simulink model "EV_model_TEMPLATE_2025a"  (R2025a)
settings: Solver=FixedStepAuto  StartTime=0.0  StopTime=1180  FixedStep=0.1  MaxStep=1e-3  RelTol=1e-3
values from neighbouring files (symbols this model uses):
  A = 2.3750    (= 2.375)    [EV_parameters.m]
  Cd = 0.24    [EV_parameters.m]
  Cr = 0.01    [EV_parameters.m]
  g = 9.81    [EV_parameters.m]
  gear_r = 9.6    [EV_parameters.m]
  grad = cos(theta)    [EV_parameters.m]
  m = 2000    [EV_parameters.m]    (also in brakes.m = 18000; powergraph.m = 18000)
  Np = 100    [EV_parameters.m]
  Ns = 100    [EV_parameters.m]
  P_max = 70    [EV_parameters.m]
  rho = 1.225    [EV_parameters.m]
  Ro = 0.07    [Battery_parameters.m]    (also in EV_parameters.m = 0.03)
  Rw = 0.35    [EV_parameters.m]
  T_max = 400    [EV_parameters.m]
  theta = 0.312    [Calculations.m]    (also in EV_parameters.m = 0)
  Voc = 3    [EV_parameters.m]
libraries: autolibshared x1, drivingcycle_lib x1, simulink x1
settings Model: Creator=Ashwil Augustin  LastModifiedBy=91944
settings SolverCC: AlgebraicLoopSolver=TrustRegion
settings DataIOCC: ReturnWorkspaceOutputs=off
settings DebuggingCC: UnconnectedInputMsg=warning  UnconnectedOutputMsg=warning  UnconnectedLineMsg=warning  PregeneratedLibrarySubsystemCodeDiagnostic=none  ArithmeticOperatorsInVariantConditions=warning
settings ModelReferenceCC: EnableRefExpFcnMdlSchedulingChecks=on
settings SFSimCC: SimUseLocalCustomCode=off  CustomCodeUndefinedFunction=UseInterfaceOnly
settings RTWCC: RTWUseLocalCustomCode=off  GPUComputeCapability=3.5  DLArmComputeVersion=19.05

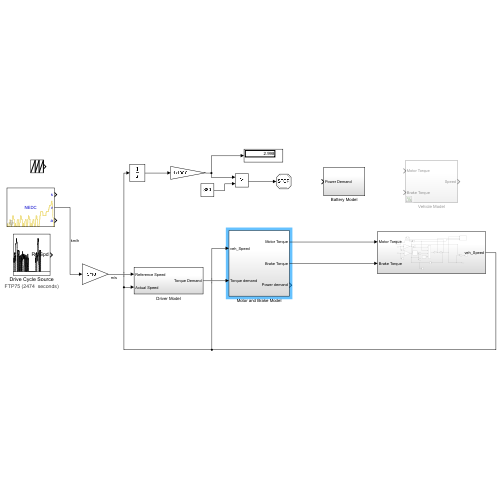
[thumbnail: Simulink's stored preview of the top-level diagram]
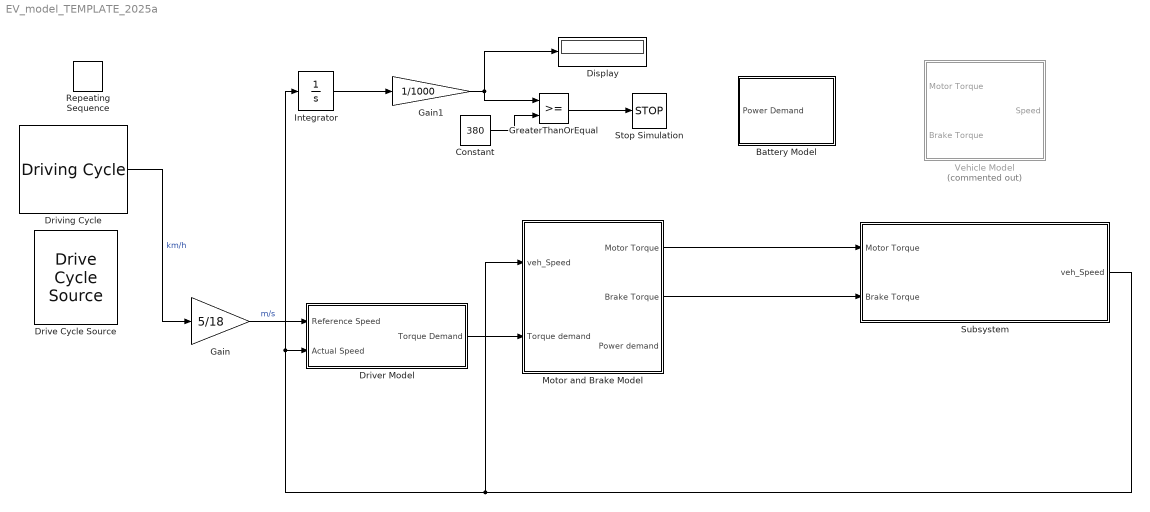
== system EV_model_TEMPLATE_2025a ==
  Battery Model : Subsystem
  Constant : Constant  Value=380
  Display : Display
  Drive Cycle Source : autolibshared/Drive Cycle Source  cycleVar=FTP75  fileVar=cycleFTP75.mat  tfinal="2474  seconds"  cycleRepeat=off  outAccPort=off  outGearPort=off  gearList=No gear data  t_wot1=5  xdot_woto=0  xdot_wot1=30  t_wot2=20  xdot_wot2=0  t_wotend=30  srcUnit=m/s  outUnit=m/s  srcAccUnit=m/s/s  outAccUnit=m/s^2  dt=0  aMode=2  faultOption=off  velBnd=2  velBndUnit=mph  inUnit=m/s  timeBnd=1  failOption=off  stopSim=off  maxFaultCnt=10  maxFaultTime=2  maxTotFaultTime=15  traceOption=off  dtTrace=1  traceWindow=10  lastDCname=FTP75  lastOutUnit=mph  lastDT=0  lastTB=1  lastSB=2  forceCalcBound=off
      settings: LibrarySourceBlock=vehdynlibscenario/Drive Cycle Source
  Driver Model : Subsystem
  Driving Cycle : drivingcycle_lib/Driving Cycle  CycleName=NEDC  CycleRepeatsForever=on
      settings: SourceProductName=Driving Cycle Blockset
  Gain : Gain  Gain=5/18
  Gain1 : Gain  Gain=1/1000
  GreaterThanOrEqual : RelationalOperator  OutDataTypeStr=boolean  RndMeth=Simplest  InputSameDT=off
  Integrator : Integrator
  Motor and Brake Model : Subsystem
  Repeating Sequence : simulink/Sources/Repeating Sequence  rep_seq_t=[0 2]  rep_seq_y=[0 2]
  Stop Simulation : Stop
  Subsystem : Subsystem
  Vehicle Model : Subsystem  Commented=on
  wires:
  Motor and Brake Model/1(Motor Torque) -> Subsystem/1("Motor Torque ")
  Driver Model/1(Torque Demand) -> Motor and Brake Model/2(Torque demand)
  Subsystem/1(veh_Speed) -> Motor and Brake Model/1(veh_Speed), Integrator/1, Driver Model/2(Actual Speed)
  Motor and Brake Model/2(Brake Torque) -> Subsystem/2(Brake Torque)
  Driving Cycle/2 -> Gain/1  "km/h"
  Gain/1 -> Driver Model/1(Reference Speed)  "m/s"
  Integrator/1 -> Gain1/1
  Constant/1 -> GreaterThanOrEqual/2
  GreaterThanOrEqual/1 -> Stop Simulation/1
  Gain1/1 -> GreaterThanOrEqual/1, Display/1

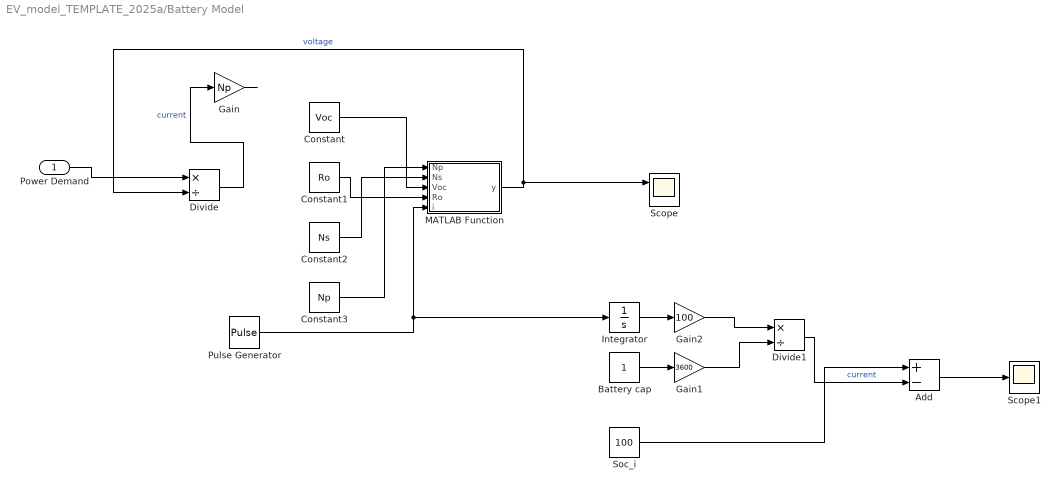
== system EV_model_TEMPLATE_2025a/Battery Model ==
  Power Demand : Inport
  Add : Sum  Inputs=+-
  Battery cap : Constant
  Constant : Constant  Value=Voc
  Constant1 : Constant  Value=Ro
  Constant2 : Constant  Value=Ns
  Constant3 : Constant  Value=Np
  Divide : Product  Inputs=*/
  Divide1 : Product  Inputs=*/
  Gain : Gain  Gain=Np
  Gain1 : Gain  Gain=3600
  Gain2 : Gain  Gain=100
  Integrator : Integrator
  MATLAB Function : MATLAB Function  TreatAsAtomicUnit=on
  Pulse Generator : DiscretePulseGenerator  PulseType=Time based  Period=10  PulseWidth=5
  Scope : Scope  NumInputPorts=2
      settings: ActiveDisplayYMinimum=2.96625  ActiveDisplayYMaximum=3.00375  DataLoggingVariableName=ScopeData2
  Scope1 : Scope
      settings: ActiveDisplayYMinimum=99.900032517604046  ActiveDisplayYMaximum=100.11119248089466  DataLoggingVariableName=ScopeData5
  Soc_i : Constant  Value=100
  wires:
  Constant3/1 -> MATLAB Function/1(Np)
  Constant2/1 -> MATLAB Function/2(Ns)
  Constant1/1 -> MATLAB Function/4(Ro)
  Constant/1 -> MATLAB Function/3(Voc)
  MATLAB Function/1(y) -> Divide/2, Scope/1  "voltage"
  Power Demand/1 -> Divide/1
  Divide/1 -> Gain/1  "current"
  Gain/1 -> ?
  Integrator/1 -> Gain2/1
  Battery cap/1 -> Gain1/1
  Gain2/1 -> Divide1/1
  Gain1/1 -> Divide1/2
  Soc_i/1 -> Add/1
  Divide1/1 -> Add/2  "current"
  Add/1 -> Scope1/1
  Pulse Generator/1 -> Integrator/1, MATLAB Function/5(i)

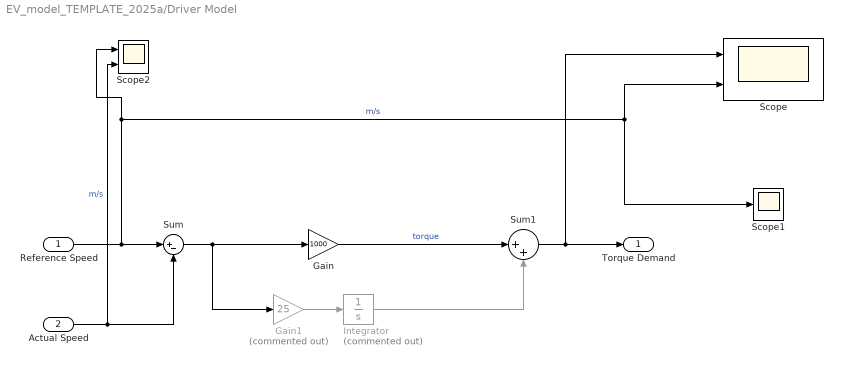
== system EV_model_TEMPLATE_2025a/Driver Model ==
  Reference Speed : Inport
  Actual Speed : Inport  Port=2
  Gain : Gain  Gain=1000
  Gain1 : Gain  Commented=on  Gain=25
  Integrator : Integrator  Commented=on
  Scope : Scope  NumInputPorts=2
      settings: ActiveDisplayYMinimum=-9.488488226261536  ActiveDisplayYMaximum=85.39639403635384  DataLoggingVariableName=ScopeData7
  Scope1 : Scope
      settings: ActiveDisplayYMinimum=-1  ActiveDisplayYMaximum=1  DataLoggingVariableName=ScopeData14
  Scope2 : Scope  NumInputPorts=2
      settings: ActiveDisplayYMinimum=3.7832627004980979  ActiveDisplayYMaximum=3.895862810225073  DataLoggingVariableName=ScopeData15
  Sum : Sum  Inputs=|+-
  Sum1 : Sum  Inputs=|++
  Torque Demand : Outport  VectorParamsAs1DForOutWhenUnconnected=off
  wires:
  Reference Speed/1 -> Scope2/1, Scope1/1, Scope/2, Sum/1  "m/s"
  Actual Speed/1 -> Scope2/2, Sum/2  "m/s"
  Sum/1 -> Gain1/1, Gain/1
  Gain/1 -> Sum1/1  "torque"
  Sum1/1 -> Scope/1, Torque Demand/1
  Integrator/1 -> Sum1/2
  Gain1/1 -> Integrator/1

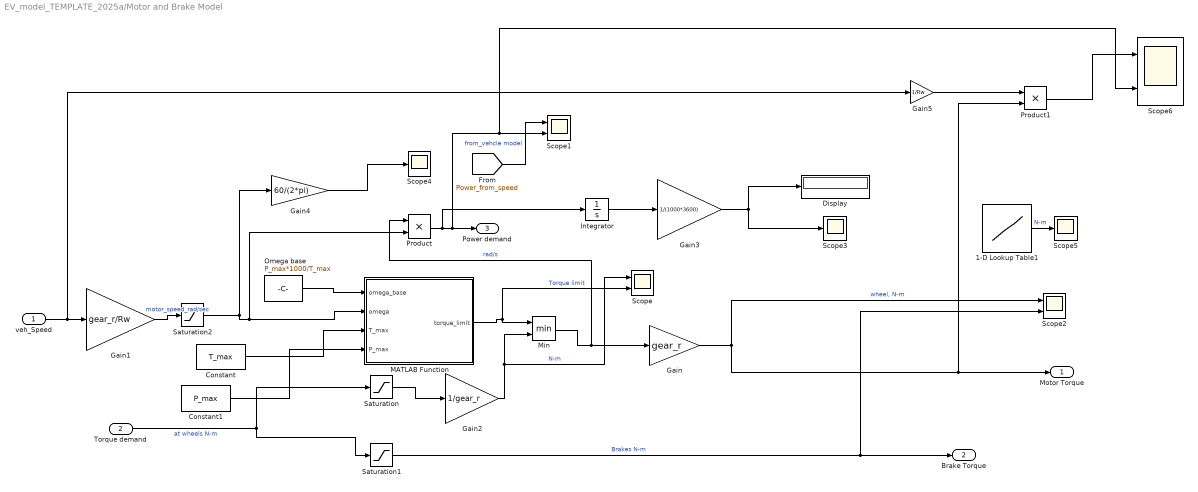
== system EV_model_TEMPLATE_2025a/Motor and Brake Model ==
  veh_Speed : Inport
  Torque demand : Inport  Port=2
  1-D Lookup Table1 : Lookup_n-D  NumberOfTableDimensions=1  BreakpointsForDimension1=[0,0.5*(70000/400), (70000/400), 2*(70000/400), 3*70000/400, 4*70000/400 ]  Table=[400,400, 400, 400/2, 400/3, 400/4]  InternalRulePriority=Speed  RndMeth=Simplest
  Constant : Constant  Value=T_max
  Constant1 : Constant  Value=P_max
  Display : Display
  Gain : Gain  Gain=gear_r
  Gain1 : Gain  Gain=gear_r/Rw
  Gain2 : Gain  Gain=1/gear_r
  Gain3 : Gain  Gain=1/(1000*3600)
  Gain4 : Gain  Gain=60/(2*pi)
  Gain5 : Gain  Gain=1/Rw
  Integrator : Integrator
  MATLAB Function : MATLAB Function  TreatAsAtomicUnit=on
  Min : MinMax  Inputs=2
  Omega base : Constant  Value=P_max*1000/T_max
  Product : Product
  Product1 : Product
  Saturation : Saturate  UpperLimit=inf  LowerLimit=0
  Saturation1 : Saturate  UpperLimit=0  LowerLimit=-inf
  Saturation2 : Saturate  UpperLimit=16000*(2*pi/60)  LowerLimit=0
  Scope{,1..2,6} (4 alike) : Scope  NumInputPorts=2
      Scope settings: ActiveDisplayYMinimum=-5.4943840804841173  ActiveDisplayYMaximum=30.78226270566185  DataLoggingVariableName=ScopeData3
      Scope1 settings: ActiveDisplayYMinimum=-7885.4073770511395  ActiveDisplayYMaximum=37796.877105105457  DataLoggingVariableName=ScopeData12
      Scope2 settings: ActiveDisplayYMinimum=-34.343817209843884  ActiveDisplayYMaximum=309.09435488859503  DataLoggingVariableName=ScopeData8
      Scope6 settings: ActiveDisplayYMinimum=-1  ActiveDisplayYMaximum=1  DataLoggingVariableName=ScopeData18
  Scope3 : Scope
      settings: ActiveDisplayYMinimum=-12.059544490137064  ActiveDisplayYMaximum=30.683168127008138  DataLoggingVariableName=ScopeData13
  Scope4 : Scope
      settings: ActiveDisplayYMinimum=-1  ActiveDisplayYMaximum=1  DataLoggingVariableName=ScopeData17
  Scope5 : Scope
      settings: ActiveDisplayYMinimum=-1  ActiveDisplayYMaximum=1  DataLoggingVariableName=ScopeData6
  Motor Torque : Outport  VectorParamsAs1DForOutWhenUnconnected=off
  Brake Torque : Outport  Port=2  VectorParamsAs1DForOutWhenUnconnected=off
  Power demand : Outport  Port=3
  wires:
  Saturation1/1 -> Scope2/2, Brake Torque/1  "Brakes N-m"
  Torque demand/1 -> Saturation/1, Saturation1/1  "at wheels N-m"
  veh_Speed/1 -> Gain5/1, Gain1/1
  Gain1/1 -> Saturation2/1  "motor_speed_rad/sec"
  Gain2/1 -> Scope/1, Min/2  "N-m"
  Saturation/1 -> Gain2/1
  Gain/1 -> Product1/2, Motor Torque/1, Scope2/1  "wheel, N-m"
  Min/1 -> Product/1, Gain/1  "rad/s"
  Product/1 -> Integrator/1, Scope6/2, Scope1/2, Power demand/1
  Integrator/1 -> Gain3/1
  Gain3/1 -> Scope3/1, Display/1
  Gain4/1 -> Scope4/1
  Omega base/1 -> MATLAB Function/1(omega_base)
  Constant/1 -> MATLAB Function/3(T_max)
  Constant1/1 -> MATLAB Function/4(P_max)
  MATLAB Function/1(torque_limit) -> Scope/2, Min/1  "Torque limit"
  [Power_from_speed] -> Scope1/1  "from_vehcle model"
  Saturation2/1 -> Gain4/1, Product/2, MATLAB Function/2(omega)
  1-D Lookup Table1/1 -> Scope5/1  "N-m"
  Gain5/1 -> Product1/1
  Product1/1 -> Scope6/1

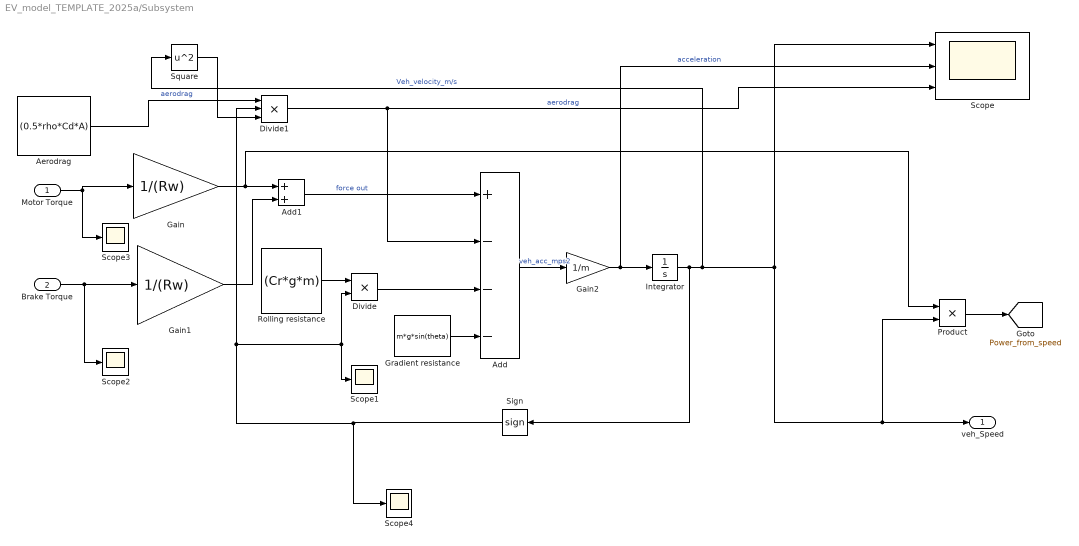
== system EV_model_TEMPLATE_2025a/Subsystem ==
  "Motor Torque " : Inport
  Brake Torque : Inport  Port=2
  Add : Sum  Inputs=+---
  Add1 : Sum
  Aerodrag : Constant  Value=(0.5*rho*Cd*A)
  Divide : Product  Inputs=**
  Divide1 : Product  Inputs=***
  Gain : Gain  Gain=1/(Rw)
  Gain1 : Gain  Gain=1/(Rw)
  Gain2 : Gain  Gain=1/m
  Gradient resistance : Constant  Value=m*g*sin(theta)
  Integrator : Integrator
  Product : Product
  Rolling resistance : Constant  Value=(Cr*g*m)
  Scope : Scope  NumInputPorts=3
      settings: ActiveDisplayYMinimum=-1.1514890830356836  ActiveDisplayYMaximum=10.328266579492118  DataLoggingVariableName=ScopeData4
  Scope{1..4} (4 alike) : Scope
      Scope1 settings: ActiveDisplayYMinimum=-0.12499999999999997  ActiveDisplayYMaximum=1.125  DataLoggingVariableName=ScopeData9
      Scope2 settings: ActiveDisplayYMinimum=-96.554250997699853  ActiveDisplayYMaximum=10.728250110855537  DataLoggingVariableName=ScopeData10
      Scope3 settings: ActiveDisplayYMinimum=-1  ActiveDisplayYMaximum=1  DataLoggingVariableName=ScopeData11
      Scope4 settings: ActiveDisplayYMinimum=-1  ActiveDisplayYMaximum=1  DataLoggingVariableName=ScopeData16
  Sign : Signum
  Square : Math  Operator=square
  veh_Speed : Outport  VectorParamsAs1DForOutWhenUnconnected=off
  tag scope: Power_from_speed=global
  wires:
  Divide1/1 -> Add/2, Scope/3  "aerodrag"
  Gain1/1 -> Add1/2
  Add/1 -> Gain2/1  "veh_acc_mps2"
  Gain/1 -> Product/1, Add1/1
  Add1/1 -> Add/1  "force out"
  Integrator/1 -> Sign/1, Square/1, Scope/1, Product/2, veh_Speed/1  "Veh_velocity_m/s"
  Aerodrag/1 -> Divide1/1  "aerodrag"
  Square/1 -> Divide1/3
  Rolling resistance/1 -> Divide/1
  "Motor Torque "/1 -> Scope3/1, Gain/1
  Divide/1 -> Add/3
  Brake Torque/1 -> Scope2/1, Gain1/1
  Sign/1 -> Scope4/1, Divide1/2, Scope1/1, Divide/2
  Gain2/1 -> Scope/2, Integrator/1  "acceleration"
  Gradient resistance/1 -> Add/4
  Product/1 -> [Power_from_speed]

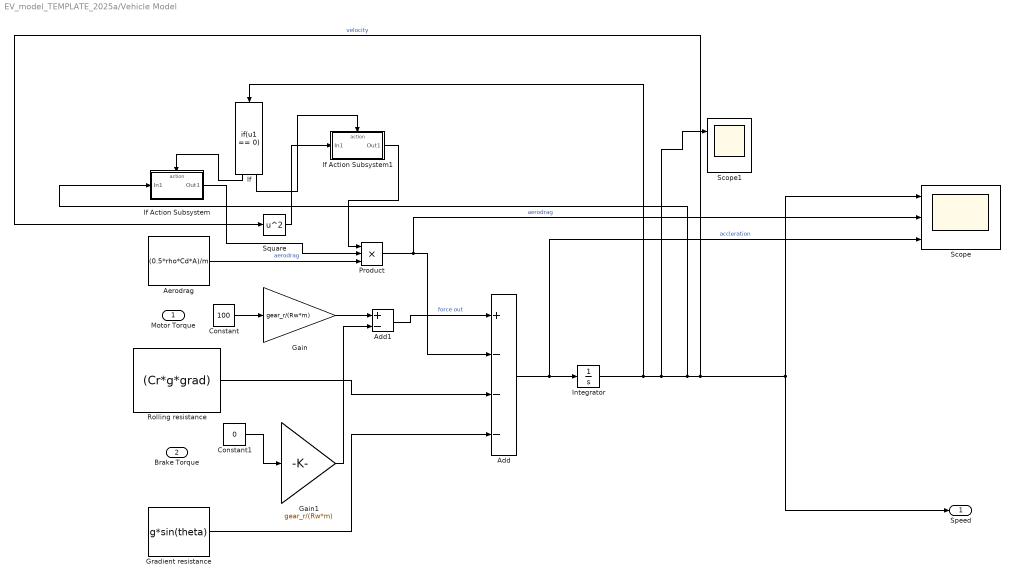
== system EV_model_TEMPLATE_2025a/Vehicle Model ==
  "Motor Torque " : Inport
  Brake Torque : Inport  Port=2
  Add : Sum  Inputs=+---
  Add1 : Sum  Inputs=+-
  Aerodrag : Constant  Value=(0.5*rho*Cd*A)/m
  Constant : Constant  Value=100
  Constant1 : Constant  Value=0
  Gain : Gain  Gain=gear_r/(Rw*m)
  Gain1 : Gain  Gain=gear_r/(Rw*m)
  Gradient resistance : Constant  Value=g*sin(theta)
  If : If  IfExpression=u1 == 0  ZeroCross=off
  If Action Subsystem : Subsystem  TreatAsAtomicUnit=on
  If Action Subsystem1 : Subsystem  TreatAsAtomicUnit=on
  Integrator : Integrator  InitialCondition=10
  Product : Product  Inputs=3
  Rolling resistance : Constant  Value=(Cr*g*grad)
  Scope : Scope  NumInputPorts=3
      settings: ActiveDisplayYMinimum=-322.61785714289488  ActiveDisplayYMaximum=3003.5607142860545
  Scope1 : Scope  NumInputPorts=2
      settings: ActiveDisplayYMinimum=3.1940786830346264  ActiveDisplayYMaximum=37.134908518455738
  Square : Math  Operator=square
  Speed : Outport  VectorParamsAs1DForOutWhenUnconnected=off
  wires:
  Rolling resistance/1 -> Add/3
  Gradient resistance/1 -> Add/4
  Add/1 -> Scope/3, Integrator/1  "accleration"
  Integrator/1 -> If/1, Scope1/1, If Action Subsystem/1(In1), Square/1, Scope/1, Speed/1  "velocity"
  Aerodrag/1 -> Product/3  "aerodrag"
  Product/1 -> Scope/2, Add/2  "aerodrag"
  Constant/1 -> Gain/1
  Gain/1 -> Add1/1
  Add1/1 -> Add/1  "force out"
  Constant1/1 -> Gain1/1
  Gain1/1 -> Add1/2
  If Action Subsystem/1(Out1) -> Product/2
  If/1 -> If Action Subsystem/Action
  If/2 -> If Action Subsystem1/Action
  Square/1 -> If Action Subsystem1/1(In1)
  If Action Subsystem1/1(Out1) -> Product/1

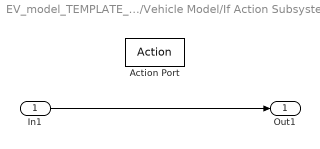
== system EV_model_TEMPLATE_2025a/Vehicle Model/If Action Subsystem ==
  In1 : Inport
  Action Port : ActionPort  ActionPortLabel=if(u1 == 0)
  Out1 : Outport
  wires:
  In1/1 -> Out1/1

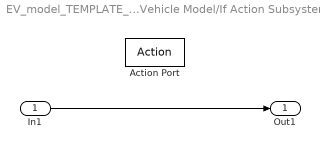
== system EV_model_TEMPLATE_2025a/Vehicle Model/If Action Subsystem1 ==
  In1 : Inport
  Action Port : ActionPort  ActionPortLabel=else
  Out1 : Outport
  wires:
  In1/1 -> Out1/1

== matlab function EV_model_TEMPLATE_2025a/Battery Model/MATLAB Function ==
  data: Np input; y output; Ns input; Voc input; Ro input; i input
function y = battery(Np, Ns, Voc,Ro,i)

y = (Ns/Np)*(Voc-i*Ro);
end

== matlab function EV_model_TEMPLATE_2025a/Motor and Brake Model/MATLAB Function ==
  data: omega_base input; omega input; torque_limit output; T_max input; P_max input
function torque_limit = fcn(omega_base, omega, T_max, P_max)

if omega <= omega_base
    torque_limit = T_max; 
else
    torque_limit = min(T_max, P_max*1000/omega);
end
